simulink model "PowerSupplySimulation"  (R2015b)
settings: Solver=ode23t  StartTime=0.0  StopTime=5*T_mach  MaxStep=1e-7  MinStep=1e-9  RelTol=1e-3
undefined symbols (not defined in the file or in its folder): c2_val, Cs, delay_load, delayVC, den_c1, den_c2, duty_inv, duty_load, f_sw, I_ref, l1_val, l2_val, num_c1, num_c2, r_val, rc2_val, rl1_val, rl2_val, Rs, t2, T_mach, V_ref, Vd_val
libraries: powerlib x64, simulink x10, simulink_extras x6, powerlib_meascontrol x5
settings Model: Creator=Akshay  LastModifiedBy=Akshay
settings SolverCC: ZeroCrossAlgorithm=Adaptive
settings DataIOCC: SaveFormat=StructureWithTime
settings HardwareCC: ProdWordSize=32  ProdHWDeviceType=Specified

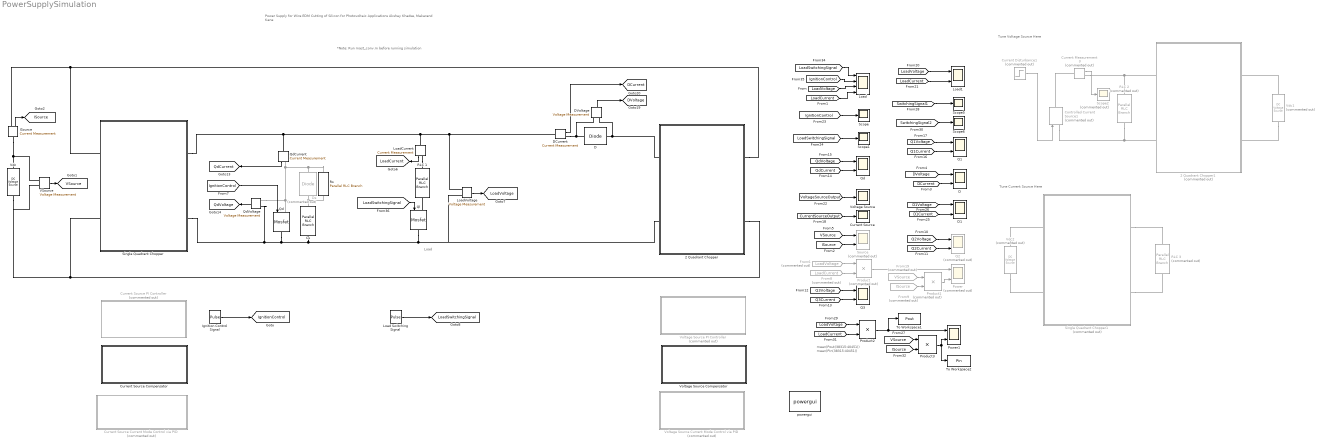
== system PowerSupplySimulation ==
  note: mean(Pout(38315:40451))
      | mean(Pin(38315:40451))
  note: Tune Current Source Here
  note: Tune Voltage Source Here
  note: Power Supply for Wire EDM Cutting of Silicon for Photovoltaic Applications
      |
      | Akshay Khadse, Makarand Kane
  note: Load
  note: *Note: Run mast_conv.m before running simulation
  " RLC 1" : powerlib/Elements/Parallel RLC Branch  LConnTagsString=a  RConnTagsString=__new0  BranchType=R  Resistance=r_val  Inductance=1e-3  SetiL0=off  InitialCurrent=0  Capacitance=0.1e-6  Setx0=off  InitialVoltage=0  Measurements=None
  " RLC 2" : powerlib/Elements/Parallel RLC Branch  Commented=on  LConnTagsString=a  RConnTagsString=__new0  BranchType=R  Resistance=r_val  Inductance=1e-3  SetiL0=off  InitialCurrent=0  Capacitance=0.1e-6  Setx0=off  InitialVoltage=0  Measurements=None
  " RLC 3" : powerlib/Elements/Parallel RLC Branch  Commented=on  LConnTagsString=a  RConnTagsString=__new0  BranchType=R  Resistance=r_val  Inductance=1e-3  SetiL0=off  InitialCurrent=0  Capacitance=0.1e-6  Setx0=off  InitialVoltage=0  Measurements=None
  " Rs" : powerlib/Elements/Parallel RLC Branch  LConnTagsString=a  RConnTagsString=__new0  BranchType=R  Resistance=Rs  Inductance=1e-3  SetiL0=off  InitialCurrent=0  Capacitance=0.1e-6  Setx0=off  InitialVoltage=0  Measurements=None
  2 Quadrant Chopper : Subsystem
  2 Quadrant Chopper1 : Subsystem  Commented=on
  Controlled Current Source1 : powerlib/Electrical Sources/Controlled Current Source  Commented=on  Initialize=on  Source_Type=AC  Amplitude=0  Phase=0  Frequency=0  Measurements=None
  Cs : powerlib/Elements/Parallel RLC Branch  LConnTagsString=a  RConnTagsString=__new0  BranchType=C  Resistance=r_val  Inductance=1e-3  SetiL0=off  InitialCurrent=0  Capacitance=Cs  Setx0=off  InitialVoltage=0  Measurements=None
  Current Disturbance1 : Step  Commented=on  Time=1e-3  After=10  SampleTime=0
  Current Measurement3 : powerlib/Measurements/Current Measurement  Commented=on  PhasorSimulation=off  OutputType=Complex  PSBequivalent=0
  Current Source : Scope
  Current Source Compensator : Subsystem
  Current Source Current Mode Control via PID : Subsystem  Commented=on
  Current Source PI Controller : Subsystem  Commented=on
  D : powerlib/Power Electronics/Diode  Ron=0.001  Lon=0  Vf=0.8  IC=0  UseSnubber=off  Rs=500  Cs=250e-9  Measurements=off
  "D " : Scope  NumInputPorts=2
  D1 : Scope  NumInputPorts=2
  DCurrent : powerlib/Measurements/Current Measurement  PhasorSimulation=off  OutputType=Complex  PSBequivalent=0
  DVoltage : powerlib/Measurements/Voltage Measurement  PhasorSimulation=off  OutputType=Complex  PSBequivalent=0
  Ds : powerlib/Power Electronics/Diode  Commented=on  Ron=0.001  Lon=0  Vf=0.8  IC=0  UseSnubber=off  Rs=500  Cs=250e-9  Measurements=off
  From19 : From  Commented=on  GotoTag=VSource  TagVisibility=global
  From6 : From  Commented=on  GotoTag=LoadVoltage  TagVisibility=global
  From8 : From  Commented=on  GotoTag=LoadCurrent  TagVisibility=global
  From9 : From  Commented=on  GotoTag=ISource  TagVisibility=global
  ISource : powerlib/Measurements/Current Measurement  PhasorSimulation=off  OutputType=Complex  PSBequivalent=0
  Ignition Control Signal : DiscretePulseGenerator  PulseType=Time based  Period=T_mach  PulseWidth=duty_inv  PhaseDelay=t2 + delayVC
  Load : Scope  NumInputPorts=4
  Load Switching Signal : DiscretePulseGenerator  PulseType=Time based  Period=T_mach  PulseWidth=duty_load  PhaseDelay=delay_load + delayVC
  Load1 : Scope  NumInputPorts=2
  LoadCurrent : powerlib/Measurements/Current Measurement  PhasorSimulation=off  OutputType=Complex  PSBequivalent=0
  LoadVoltage : powerlib/Measurements/Voltage Measurement  PhasorSimulation=off  OutputType=Complex  PSBequivalent=0
  Power : Scope  Commented=on  NumInputPorts=2
  Power1 : Scope  NumInputPorts=2
  Product : Product  Commented=on
  Product1 : Product  Commented=on
  Product2 : Product
  Product3 : Product
  "Q1 " : Scope  NumInputPorts=2
  "Q2 " : Scope  Commented=on  NumInputPorts=2
  "Q3 " : Scope  NumInputPorts=2
  Qd : powerlib/Power Electronics/Mosfet  Ron=0.1  Lon=0  Rd=0.01  Vfd=0  IC=0  Rs=1e5  Cs=inf  Measurements=off
  "Qd " : Scope  NumInputPorts=2
  QdCurrent : powerlib/Measurements/Current Measurement  PhasorSimulation=off  OutputType=Complex  PSBequivalent=0
  QdVoltage : powerlib/Measurements/Voltage Measurement  PhasorSimulation=off  OutputType=Complex  PSBequivalent=0
  Ql : powerlib/Power Electronics/Mosfet  Ron=0.1  Lon=0  Rd=0.01  Vfd=0  IC=0  Rs=1e5  Cs=inf  Measurements=off
  Scope{,1,5..6} (4 alike) : Scope
  Scope2 : Scope  Commented=on
  Single Quadrant Chopper : Subsystem
  Single Quadrant Chopper1 : Subsystem  Commented=on
  Source : Scope  Commented=on  NumInputPorts=2
  To Workspace1 : ToWorkspace  VariableName=Pout  SampleTime=-1
  To Workspace2 : ToWorkspace  VariableName=Pin  SampleTime=-1
  VSource : powerlib/Measurements/Voltage Measurement  PhasorSimulation=off  OutputType=Complex  PSBequivalent=0
  Vdc : powerlib/Electrical Sources/DC Voltage Source  Amplitude=Vd_val  Measurements=Voltage
  Vdc1 : powerlib/Electrical Sources/DC Voltage Source  Commented=on  Amplitude=Vd_val  Measurements=Voltage
  Vdc2 : powerlib/Electrical Sources/DC Voltage Source  Commented=on  Amplitude=Vd_val  Measurements=Voltage
  Voltage Source : Scope
  Voltage Source Compensator : Subsystem
  Voltage Source Current Mode Control via PID : Subsystem  Commented=on
  Voltage Source PI Controller : Subsystem  Commented=on
  powergui : powerlib/powergui  Priority=1  SimulationMode=Continuous  SolverType=Backward Euler  SampleTime=5e-07  frequency=60  SPID=on  DisableSnubberDevices=off  DisableRonSwitches=off  DisableVfSwitches=off  SwTol=0  DisplayEquations=off  Interpol=off  ExternalGateDelay=off  methode=off  Ts=0  FunctionMessages=off  echomessages=off  HookPort=off  EnableUseOfTLC=off  x0status=zero  frequencyindice=0  Pbase=100e6  ErrMax=1e-4  Iterations=50  UnitsV=kV  UnitsW=MW  buscounter=0  RestoreLinks=warning  ResistiveCurrentMeasurement=off  Frange=[0:2:500]  Ylog=off  Xlog=on  ShowGrid=off  save=off  variable=ZData  structure=ScopeData  ZoomFFT=off  StartTime=0.0  cycles=5  DisplayStyle=2  fundamental=50  FreqAxis=off  MaxFrequency=50000  frequencyindicesteady=1  RmsSteady=1  display=off
  tag scope: DCurrent=global, DVoltage=global, ISource=global, IgnitionControl=global, LoadCurrent=global, LoadSwitchingSignal=global, LoadVoltage=global, QdCurrent=global, QdVoltage=global, VSource=global
  wires:
  Ignition Control Signal/1 -> [IgnitionControl]
  Load Switching Signal/1 -> [LoadSwitchingSignal]
  [Q2Voltage] -> "Q2 "/1
  [Q2Current] -> "Q2 "/2
  [Q1Voltage] -> "Q1 "/1
  [Q1Current] -> "Q1 "/2
  [QdVoltage] -> "Qd "/1
  [QdCurrent] -> "Qd "/2
  [VoltageSourceOutput] -> Voltage Source/1
  [IgnitionControl] -> Scope/1
  [LoadSwitchingSignal] -> Scope1/1
  [CurrentSourceOutput] -> Current Source/1
  LoadCurrent/1 -> [LoadCurrent]
  LoadVoltage/1 -> [LoadVoltage]
  [IgnitionControl] -> Qd/1
  QdCurrent/1 -> [QdCurrent]
  QdVoltage/1 -> [QdVoltage]
  DVoltage/1 -> [DVoltage]
  DCurrent/1 -> [DCurrent]
  [LoadSwitchingSignal] -> Load/1
  [IgnitionControl] -> Load/2
  [LoadVoltage] -> Load/3
  [LoadCurrent] -> Load/4
  [LoadSwitchingSignal] -> Ql/1
  [SwitchingSignal2] -> Scope6/1
  [SwitchingSignal1] -> Scope5/1
  [DVoltage] -> "D "/1
  [DCurrent] -> "D "/2
  VSource/1 -> [VSource]
  ISource/1 -> [ISource]
  [VSource] -> Source/1
  [ISource] -> Source/2
  From6/1 -> Product/1
  From8/1 -> Product/2
  From19/1 -> Product1/1
  From9/1 -> Product1/2
  Product/1 -> Power/1
  Product1/1 -> Power/2
  [D1Voltage] -> D1/1
  [D1Current] -> D1/2
  Current Disturbance1/1 -> Controlled Current Source1/1
  Current Measurement3/1 -> Scope2/1
  [LoadVoltage] -> Load1/1
  [LoadCurrent] -> Load1/2
  [Q3Voltage] -> "Q3 "/1
  [Q3Current] -> "Q3 "/2
  [LoadVoltage] -> Product2/1
  [LoadCurrent] -> Product2/2
  [VSource] -> Product3/1
  [ISource] -> Product3/2
  Product2/1 -> To Workspace1/1, Power1/1
  Product3/1 -> Power1/2, To Workspace2/1
  connections:
  LoadCurrent/RConn1 -- " RLC 1"/LConn1
  Ds/LConn1 -- QdVoltage/LConn1 -- Qd/LConn1 -- QdCurrent/RConn1 -- " Rs"/LConn1
  DVoltage/LConn1 -- DCurrent/RConn1 -- D/LConn1
  DCurrent/LConn1 -- LoadVoltage/LConn1 -- LoadCurrent/LConn1 -- QdCurrent/LConn1 -- Single Quadrant Chopper/RConn1
  2 Quadrant Chopper/RConn1 -- ISource/RConn1 -- Single Quadrant Chopper/LConn1
  2 Quadrant Chopper/RConn2 -- VSource/LConn2 -- Vdc/LConn1 -- Single Quadrant Chopper/LConn2
  Ql/LConn1 -- " RLC 1"/RConn1
  D/RConn1 -- 2 Quadrant Chopper/LConn1 -- DVoltage/LConn2
  Qd/RConn1 -- 2 Quadrant Chopper/LConn2 -- LoadVoltage/LConn2 -- Ql/RConn1 -- Cs/RConn1 -- QdVoltage/LConn2 -- Single Quadrant Chopper/RConn2
  ISource/LConn1 -- Vdc/RConn1 -- VSource/LConn1
  " RLC 2"/LConn1 -- Current Measurement3/RConn1 -- 2 Quadrant Chopper1/LConn1
  " RLC 2"/RConn1 -- Controlled Current Source1/LConn1 -- 2 Quadrant Chopper1/LConn2
  Vdc1/RConn1 -- 2 Quadrant Chopper1/RConn1
  Vdc1/LConn1 -- 2 Quadrant Chopper1/RConn2
  Vdc2/RConn1 -- Single Quadrant Chopper1/LConn1
  Vdc2/LConn1 -- Single Quadrant Chopper1/LConn2
  Single Quadrant Chopper1/RConn1 -- " RLC 3"/LConn1
  Single Quadrant Chopper1/RConn2 -- " RLC 3"/RConn1
  Ds/RConn1 -- " Rs"/RConn1 -- Cs/LConn1
  Controlled Current Source1/RConn1 -- Current Measurement3/LConn1

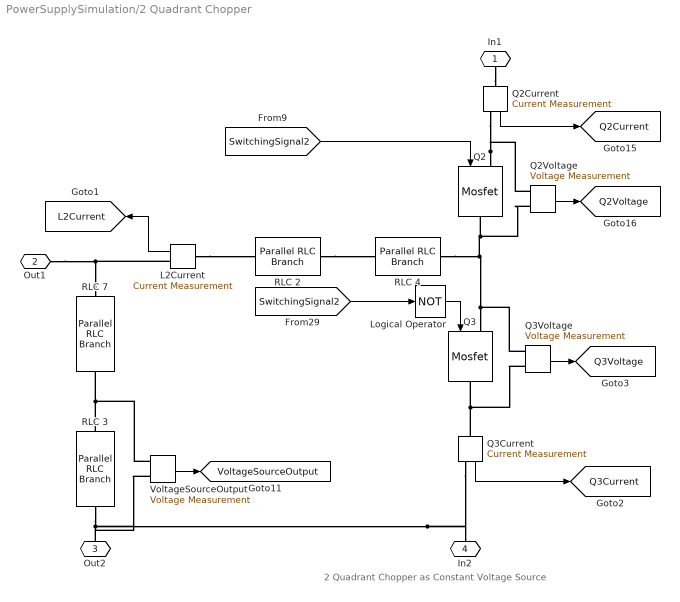
== system PowerSupplySimulation/2 Quadrant Chopper ==
  note: 2 Quadrant Chopper as Constant Voltage Source
  " RLC 2" : powerlib/Elements/Parallel RLC Branch  LConnTagsString=a  RConnTagsString=__new0  BranchType=R  Resistance=rl2_val  Inductance=5e-6  SetiL0=off  InitialCurrent=0  Capacitance=0.3e-6  Setx0=off  InitialVoltage=0  Measurements=None
  " RLC 3" : powerlib/Elements/Parallel RLC Branch  LConnTagsString=a  RConnTagsString=__new0  BranchType=C  Resistance=1  Inductance=1e-3  SetiL0=off  InitialCurrent=0  Capacitance=c2_val  Setx0=off  InitialVoltage=50  Measurements=None
  " RLC 4" : powerlib/Elements/Parallel RLC Branch  LConnTagsString=a  RConnTagsString=__new0  BranchType=L  Resistance=50  Inductance=l2_val  SetiL0=off  InitialCurrent=0  Capacitance=0.3e-6  Setx0=off  InitialVoltage=0  Measurements=None
  " RLC 7" : powerlib/Elements/Parallel RLC Branch  LConnTagsString=a  RConnTagsString=__new0  BranchType=R  Resistance=rc2_val  Inductance=1e-3  SetiL0=off  InitialCurrent=0  Capacitance=0.1e-6  Setx0=off  InitialVoltage=0  Measurements=None
  L2Current : powerlib/Measurements/Current Measurement  PhasorSimulation=off  OutputType=Complex  PSBequivalent=0
  Logical Operator : Logic  Operator=NOT  AllPortsSameDT=off  OutDataTypeStr=boolean
  Q2 : powerlib/Power Electronics/Mosfet  Ron=0.1  Lon=0  Rd=0.01  Vfd=0  IC=0  Rs=1e5  Cs=inf  Measurements=off
  Q2Current : powerlib/Measurements/Current Measurement  PhasorSimulation=off  OutputType=Complex  PSBequivalent=0
  Q2Voltage : powerlib/Measurements/Voltage Measurement  PhasorSimulation=off  OutputType=Complex  PSBequivalent=0
  Q3 : powerlib/Power Electronics/Mosfet  Ron=0.1  Lon=0  Rd=0.01  Vfd=0  IC=0  Rs=1e5  Cs=inf  Measurements=off
  Q3Current : powerlib/Measurements/Current Measurement  PhasorSimulation=off  OutputType=Complex  PSBequivalent=0
  Q3Voltage : powerlib/Measurements/Voltage Measurement  PhasorSimulation=off  OutputType=Complex  PSBequivalent=0
  VoltageSourceOutput : powerlib/Measurements/Voltage Measurement  PhasorSimulation=off  OutputType=Complex  PSBequivalent=0
  In1 : PMIOPort  Port=1  Side=Right
  Out1 : PMIOPort  Port=2  Side=Left
  Out2 : PMIOPort  Port=3  Side=Left
  In2 : PMIOPort  Port=4  Side=Right
  tag scope: L2Current=global, Q2Current=global, Q2Voltage=global, Q3Current=global, Q3Voltage=global, VoltageSourceOutput=global
  wires:
  Logical Operator/1 -> Q3/1
  VoltageSourceOutput/1 -> [VoltageSourceOutput]
  Q3Current/1 -> [Q3Current]
  Q3Voltage/1 -> [Q3Voltage]
  Q2Voltage/1 -> [Q2Voltage]
  Q2Current/1 -> [Q2Current]
  [SwitchingSignal2] -> Q2/1
  [SwitchingSignal2] -> Logical Operator/1
  L2Current/1 -> [L2Current]
  connections:
  " RLC 3"/RConn1 -- VoltageSourceOutput/LConn2 -- Q3Current/RConn1 -- In2/RConn1 -- Out2/RConn1
  VoltageSourceOutput/LConn1 -- " RLC 3"/LConn1 -- " RLC 7"/RConn1
  Q3Voltage/LConn2 -- Q3Current/LConn1 -- Q3/RConn1
  Q2/LConn1 -- Q2Voltage/LConn1 -- Q2Current/RConn1
  " RLC 2"/RConn1 -- " RLC 4"/LConn1
  In1/RConn1 -- Q2Current/LConn1
  Out1/RConn1 -- L2Current/RConn1 -- " RLC 7"/LConn1
  " RLC 4"/RConn1 -- Q3Voltage/LConn1 -- Q3/LConn1 -- Q2Voltage/LConn2 -- Q2/RConn1
  L2Current/LConn1 -- " RLC 2"/LConn1

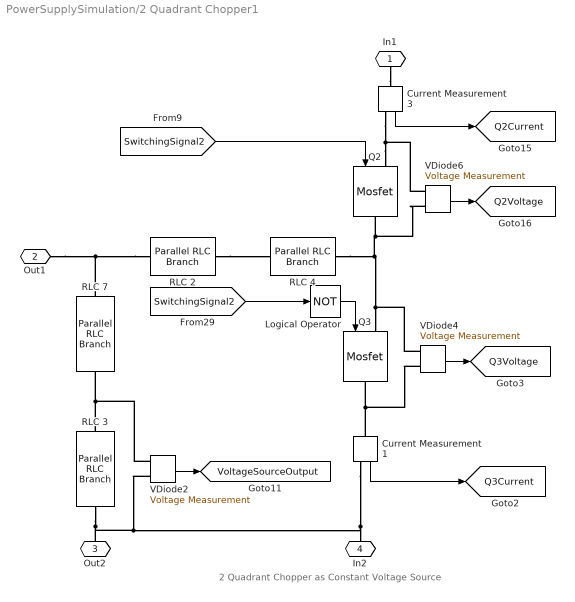
== system PowerSupplySimulation/2 Quadrant Chopper1 ==
  note: 2 Quadrant Chopper as Constant Voltage Source
  " RLC 2" : powerlib/Elements/Parallel RLC Branch  LConnTagsString=a  RConnTagsString=__new0  BranchType=R  Resistance=rl2_val  Inductance=5e-6  SetiL0=off  InitialCurrent=0  Capacitance=0.3e-6  Setx0=off  InitialVoltage=0  Measurements=None
  " RLC 3" : powerlib/Elements/Parallel RLC Branch  LConnTagsString=a  RConnTagsString=__new0  BranchType=C  Resistance=1  Inductance=1e-3  SetiL0=off  InitialCurrent=0  Capacitance=c2_val  Setx0=off  InitialVoltage=50  Measurements=None
  " RLC 4" : powerlib/Elements/Parallel RLC Branch  LConnTagsString=a  RConnTagsString=__new0  BranchType=L  Resistance=50  Inductance=l2_val  SetiL0=off  InitialCurrent=0  Capacitance=0.3e-6  Setx0=off  InitialVoltage=0  Measurements=None
  " RLC 7" : powerlib/Elements/Parallel RLC Branch  LConnTagsString=a  RConnTagsString=__new0  BranchType=R  Resistance=rc2_val  Inductance=1e-3  SetiL0=off  InitialCurrent=0  Capacitance=0.1e-6  Setx0=off  InitialVoltage=0  Measurements=None
  Current Measurement1 : powerlib/Measurements/Current Measurement  PhasorSimulation=off  OutputType=Complex  PSBequivalent=0
  Current Measurement3 : powerlib/Measurements/Current Measurement  PhasorSimulation=off  OutputType=Complex  PSBequivalent=0
  Logical Operator : Logic  Operator=NOT  AllPortsSameDT=off  OutDataTypeStr=boolean
  Q2 : powerlib/Power Electronics/Mosfet  Ron=0.1  Lon=0  Rd=0.01  Vfd=0  IC=0  Rs=1e5  Cs=inf  Measurements=off
  Q3 : powerlib/Power Electronics/Mosfet  Ron=0.1  Lon=0  Rd=0.01  Vfd=0  IC=0  Rs=1e5  Cs=inf  Measurements=off
  VDiode2 : powerlib/Measurements/Voltage Measurement  PhasorSimulation=off  OutputType=Complex  PSBequivalent=0
  VDiode4 : powerlib/Measurements/Voltage Measurement  PhasorSimulation=off  OutputType=Complex  PSBequivalent=0
  VDiode6 : powerlib/Measurements/Voltage Measurement  PhasorSimulation=off  OutputType=Complex  PSBequivalent=0
  In1 : PMIOPort  Port=1  Side=Right
  Out1 : PMIOPort  Port=2  Side=Left
  Out2 : PMIOPort  Port=3  Side=Left
  In2 : PMIOPort  Port=4  Side=Right
  tag scope: Q2Current=global, Q2Voltage=global, Q3Current=global, Q3Voltage=global, VoltageSourceOutput=global
  wires:
  Logical Operator/1 -> Q3/1
  VDiode2/1 -> [VoltageSourceOutput]
  Current Measurement1/1 -> [Q3Current]
  VDiode4/1 -> [Q3Voltage]
  VDiode6/1 -> [Q2Voltage]
  Current Measurement3/1 -> [Q2Current]
  [SwitchingSignal2] -> Q2/1
  [SwitchingSignal2] -> Logical Operator/1
  connections:
  " RLC 3"/RConn1 -- Current Measurement1/RConn1 -- In2/RConn1 -- VDiode2/LConn2 -- Out2/RConn1
  VDiode2/LConn1 -- " RLC 3"/LConn1 -- " RLC 7"/RConn1
  VDiode4/LConn2 -- Current Measurement1/LConn1 -- Q3/RConn1
  Q2/LConn1 -- VDiode6/LConn1 -- Current Measurement3/RConn1
  " RLC 2"/RConn1 -- " RLC 4"/LConn1
  In1/RConn1 -- Current Measurement3/LConn1
  " RLC 2"/LConn1 -- " RLC 7"/LConn1 -- Out1/RConn1
  " RLC 4"/RConn1 -- VDiode4/LConn1 -- Q3/LConn1 -- VDiode6/LConn2 -- Q2/RConn1

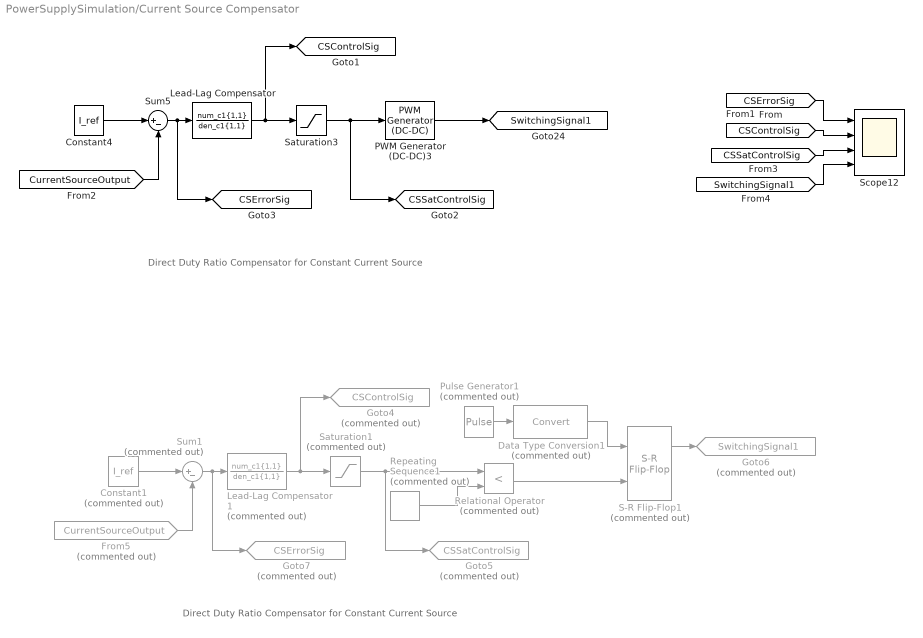
== system PowerSupplySimulation/Current Source Compensator ==
  note: Direct Duty Ratio Compensator for Constant Current Source
  note: Direct Duty Ratio Compensator for Constant Current Source
  Constant1 : Constant  Commented=on  Value=I_ref
  Constant4 : Constant  Value=I_ref
  Data Type Conversion1 : DataTypeConversion  Commented=on
  From5 : From  Commented=on  GotoTag=CurrentSourceOutput  TagVisibility=global
  Goto4 : Goto  Commented=on  GotoTag=CSControlSig  TagVisibility=global
  Goto5 : Goto  Commented=on  GotoTag=CSSatControlSig  TagVisibility=global
  Goto6 : Goto  Commented=on  GotoTag=SwitchingSignal1  TagVisibility=global
  Goto7 : Goto  Commented=on  GotoTag=CSErrorSig  TagVisibility=global
  Lead-Lag Compensator : TransferFcn  Numerator=num_c1{1,1}  Denominator=den_c1{1,1}
  Lead-Lag Compensator1 : TransferFcn  Commented=on  Numerator=num_c1{1,1}  Denominator=den_c1{1,1}
  PWM Generator (DC-DC)3 : powerlib_meascontrol/Pulse & Signal Generators/PWM Generator (DC-DC)  Fsw=f_sw  Ts=0
  Pulse Generator1 : DiscretePulseGenerator  Commented=on  PulseType=Time based  Period=1/f_sw  PulseWidth=5
  Relational Operator : RelationalOperator  Commented=on  Operator=<  OutDataTypeStr=boolean
  Repeating Sequence1 : simulink/Sources/Repeating Sequence  Commented=on  rep_seq_t=[0 1/f_sw]  rep_seq_y=[0 1]
  S-R Flip-Flop1 : simulink_extras/Flip Flops/S-R Flip-Flop  Commented=on  initial_condition=0
  Saturation1 : Saturate  Commented=on  UpperLimit=0.99  LowerLimit=0
  Saturation3 : Saturate  UpperLimit=0.99  LowerLimit=0
  Scope12 : Scope  NumInputPorts=4
  Sum1 : Sum  Commented=on  Inputs=|+-
  Sum5 : Sum  Inputs=|+-
  tag scope: CSControlSig=global, CSErrorSig=global, CSSatControlSig=global, SwitchingSignal1=global
  wires:
  Sum5/1 -> [CSErrorSig], Lead-Lag Compensator/1
  Constant4/1 -> Sum5/1
  [CurrentSourceOutput] -> Sum5/2
  Lead-Lag Compensator/1 -> Saturation3/1, [CSControlSig]
  Saturation3/1 -> [CSSatControlSig], PWM Generator (DC-DC)3/1
  PWM Generator (DC-DC)3/1 -> [SwitchingSignal1]
  [CSErrorSig] -> Scope12/1
  [CSControlSig] -> Scope12/2
  [CSSatControlSig] -> Scope12/3
  [SwitchingSignal1] -> Scope12/4
  Sum1/1 -> Goto7/1, Lead-Lag Compensator1/1
  Constant1/1 -> Sum1/1
  From5/1 -> Sum1/2
  Lead-Lag Compensator1/1 -> Saturation1/1, Goto4/1
  Saturation1/1 -> Relational Operator/1, Goto5/1
  Repeating Sequence1/1 -> Relational Operator/2
  S-R Flip-Flop1/1 -> Goto6/1
  Pulse Generator1/1 -> Data Type Conversion1/1
  Data Type Conversion1/1 -> S-R Flip-Flop1/1
  Relational Operator/1 -> S-R Flip-Flop1/2

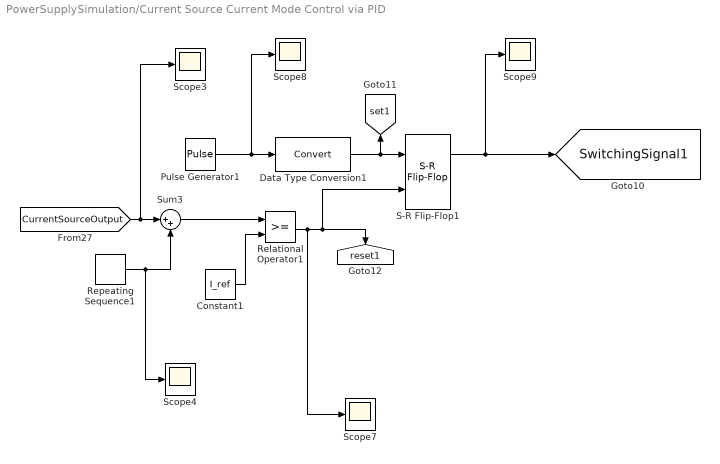
== system PowerSupplySimulation/Current Source Current Mode Control via PID ==
  Constant1 : Constant  Value=I_ref
  Data Type Conversion1 : DataTypeConversion
  Pulse Generator1 : DiscretePulseGenerator  PulseType=Time based  Period=1/f_sw  PulseWidth=5
  Relational Operator1 : RelationalOperator  OutDataTypeStr=boolean
  Repeating Sequence1 : simulink/Sources/Repeating Sequence  rep_seq_t=[0 1/f_sw]  rep_seq_y=[0 0]
  S-R Flip-Flop1 : simulink_extras/Flip Flops/S-R Flip-Flop  initial_condition=0
  Scope{3..4,7..9} (5 alike) : Scope
  Sum3 : Sum  Inputs=|++
  tag scope: SwitchingSignal1=global, reset1=global, set1=global
  wires:
  Pulse Generator1/1 -> Scope8/1, Data Type Conversion1/1
  Data Type Conversion1/1 -> S-R Flip-Flop1/1, [set1]
  Relational Operator1/1 -> Scope7/1, S-R Flip-Flop1/2, [reset1]
  S-R Flip-Flop1/1 -> Scope9/1, [SwitchingSignal1]
  [CurrentSourceOutput] -> Scope3/1, Sum3/1
  Repeating Sequence1/1 -> Scope4/1, Sum3/2
  Sum3/1 -> Relational Operator1/1
  Constant1/1 -> Relational Operator1/2

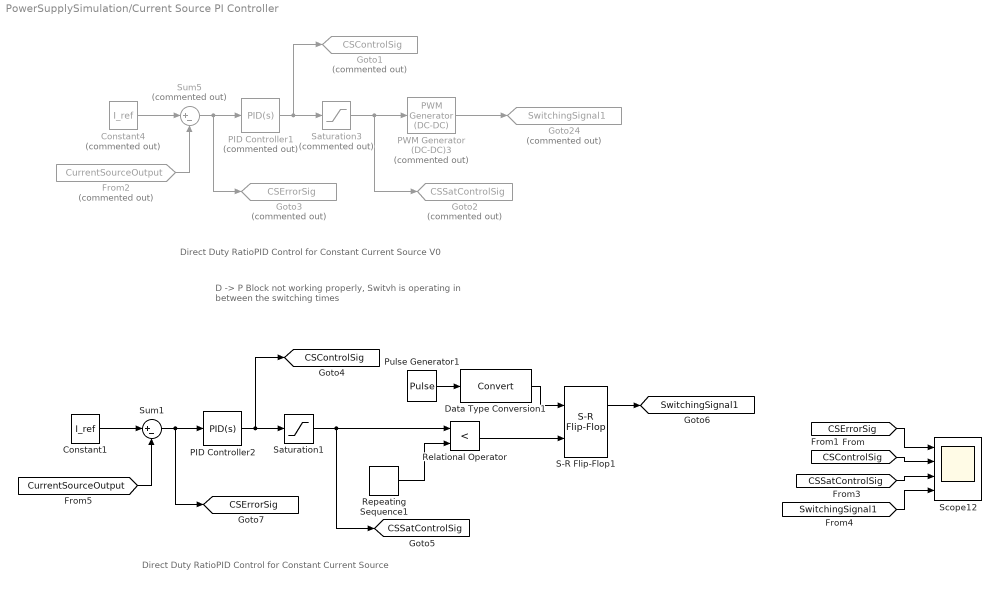
== system PowerSupplySimulation/Current Source PI Controller ==
  note: D -> P Block not working properly,
      | Switvh is operating in between the switching times
  note: Direct Duty RatioPID Control for Constant Current Source V0
  note: Direct Duty RatioPID Control for Constant Current Source
  Constant1 : Constant  Value=I_ref
  Constant4 : Constant  Commented=on  Value=I_ref
  Data Type Conversion1 : DataTypeConversion
  From2 : From  Commented=on  GotoTag=CurrentSourceOutput  TagVisibility=global
  Goto1 : Goto  Commented=on  GotoTag=CSControlSig  TagVisibility=global
  Goto2 : Goto  Commented=on  GotoTag=CSSatControlSig  TagVisibility=global
  Goto24 : Goto  Commented=on  GotoTag=SwitchingSignal1  TagVisibility=global
  Goto3 : Goto  Commented=on  GotoTag=CSErrorSig  TagVisibility=global
  PID Controller1 : simulink/Continuous/PID Controller  Commented=on  Controller=PID  TimeDomain=Continuous-time  SampleTime=-1  IntegratorMethod=Forward Euler  FilterMethod=Forward Euler  Form=Parallel  UseFilter=on  ControllerParametersSource=internal  P=3  I=0  D=0  N=5  InitialConditionSource=internal  InitialConditionForIntegrator=0  InitialConditionForFilter=0  ExternalReset=none  LimitOutput=off  UpperSaturationLimit=inf  LowerSaturationLimit=-inf  LinearizeAsGain=on  AntiWindupMode=none  Kb=1  TrackingMode=off  Kt=1  PParamMin=[]  PParamMax=[]  IParamMin=[]  IParamMax=[]  DParamMin=[]  DParamMax=[]  NParamMin=[]  NParamMax=[]  KbParamMin=[]  KbParamMax=[]  KtParamMin=[]  KtParamMax=[]  POutMin=[]  POutMax=[]  IOutMin=[]  IOutMax=[]  DOutMin=[]  DOutMax=[]  NOutMin=[]  NOutMax=[]  KbOutMin=[]  KbOutMax=[]  KtOutMin=[]  KtOutMax=[]  IntegratorOutMin=[]  IntegratorOutMax=[]  FilterOutMin=[]  FilterOutMax=[]  SumOutMin=[]  SumOutMax=[]  SumI1OutMin=[]  SumI1OutMax=[]  SumI2OutMin=[]  SumI2OutMax=[]  SumI3OutMin=[]  SumI3OutMax=[]  SumDOutMin=[]  SumDOutMax=[]  SaturationOutMin=[]  SaturationOutMax=[]  IntegratorContinuousStateAttributes=''  IntegratorStateMustResolveToSignalObject=off  IntegratorRTWStateStorageClass=Auto  FilterContinuousStateAttributes=''  FilterStateMustResolveToSignalObject=off  FilterRTWStateStorageClass=Auto  DifferentiatorICPrevScaledInput=0  DifferentiatorOutMin=[]  DifferentiatorOutMax=[]
  PID Controller2 : simulink/Continuous/PID Controller  Controller=PID  TimeDomain=Continuous-time  SampleTime=-1  IntegratorMethod=Forward Euler  FilterMethod=Forward Euler  Form=Parallel  UseFilter=on  ControllerParametersSource=internal  P=1  I=0  D=0  N=5  InitialConditionSource=internal  InitialConditionForIntegrator=0  InitialConditionForFilter=0  ExternalReset=none  LimitOutput=off  UpperSaturationLimit=inf  LowerSaturationLimit=-inf  LinearizeAsGain=on  AntiWindupMode=none  Kb=1  TrackingMode=off  Kt=1  PParamMin=[]  PParamMax=[]  IParamMin=[]  IParamMax=[]  DParamMin=[]  DParamMax=[]  NParamMin=[]  NParamMax=[]  KbParamMin=[]  KbParamMax=[]  KtParamMin=[]  KtParamMax=[]  POutMin=[]  POutMax=[]  IOutMin=[]  IOutMax=[]  DOutMin=[]  DOutMax=[]  NOutMin=[]  NOutMax=[]  KbOutMin=[]  KbOutMax=[]  KtOutMin=[]  KtOutMax=[]  IntegratorOutMin=[]  IntegratorOutMax=[]  FilterOutMin=[]  FilterOutMax=[]  SumOutMin=[]  SumOutMax=[]  SumI1OutMin=[]  SumI1OutMax=[]  SumI2OutMin=[]  SumI2OutMax=[]  SumI3OutMin=[]  SumI3OutMax=[]  SumDOutMin=[]  SumDOutMax=[]  SaturationOutMin=[]  SaturationOutMax=[]  IntegratorContinuousStateAttributes=''  IntegratorStateMustResolveToSignalObject=off  IntegratorRTWStateStorageClass=Auto  FilterContinuousStateAttributes=''  FilterStateMustResolveToSignalObject=off  FilterRTWStateStorageClass=Auto  DifferentiatorICPrevScaledInput=0  DifferentiatorOutMin=[]  DifferentiatorOutMax=[]
  PWM Generator (DC-DC)3 : powerlib_meascontrol/Pulse & Signal Generators/PWM Generator (DC-DC)  Commented=on  Fsw=f_sw  Ts=0
  Pulse Generator1 : DiscretePulseGenerator  PulseType=Time based  Period=1/f_sw  PulseWidth=5
  Relational Operator : RelationalOperator  Operator=<  OutDataTypeStr=boolean
  Repeating Sequence1 : simulink/Sources/Repeating Sequence  rep_seq_t=[0 1/f_sw]  rep_seq_y=[0 1]
  S-R Flip-Flop1 : simulink_extras/Flip Flops/S-R Flip-Flop  initial_condition=0
  Saturation1 : Saturate  UpperLimit=0.99  LowerLimit=0
  Saturation3 : Saturate  Commented=on  UpperLimit=0.99  LowerLimit=0
  Scope12 : Scope  NumInputPorts=4
  Sum1 : Sum  Inputs=|+-
  Sum5 : Sum  Commented=on  Inputs=|+-
  tag scope: CSControlSig=global, CSErrorSig=global, CSSatControlSig=global, SwitchingSignal1=global
  wires:
  Sum5/1 -> Goto3/1, PID Controller1/1
  Constant4/1 -> Sum5/1
  From2/1 -> Sum5/2
  PID Controller1/1 -> Saturation3/1, Goto1/1
  Saturation3/1 -> Goto2/1, PWM Generator (DC-DC)3/1
  PWM Generator (DC-DC)3/1 -> Goto24/1
  [CSErrorSig] -> Scope12/1
  [CSControlSig] -> Scope12/2
  [CSSatControlSig] -> Scope12/3
  [SwitchingSignal1] -> Scope12/4
  Sum1/1 -> [CSErrorSig], PID Controller2/1
  Constant1/1 -> Sum1/1
  [CurrentSourceOutput] -> Sum1/2
  PID Controller2/1 -> Saturation1/1, [CSControlSig]
  Repeating Sequence1/1 -> Relational Operator/2
  Relational Operator/1 -> S-R Flip-Flop1/2
  Saturation1/1 -> Relational Operator/1, [CSSatControlSig]
  S-R Flip-Flop1/1 -> [SwitchingSignal1]
  Data Type Conversion1/1 -> S-R Flip-Flop1/1
  Pulse Generator1/1 -> Data Type Conversion1/1

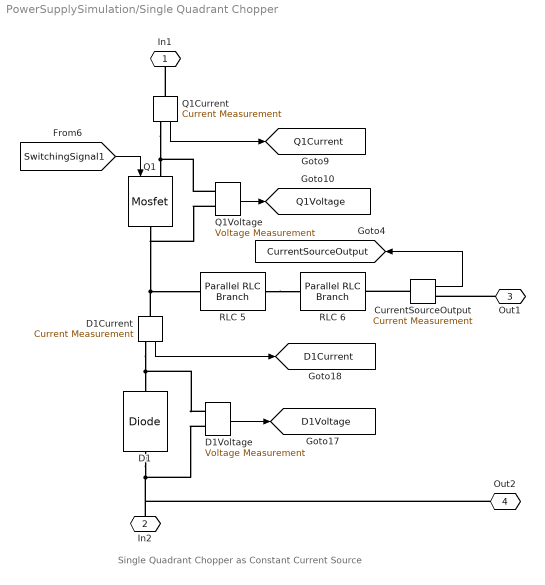
== system PowerSupplySimulation/Single Quadrant Chopper ==
  note: Single Quadrant Chopper as Constant Current Source
  " RLC 5" : powerlib/Elements/Parallel RLC Branch  LConnTagsString=a  RConnTagsString=__new0  BranchType=R  Resistance=rl1_val  Inductance=5e-6  SetiL0=off  InitialCurrent=0  Capacitance=0.3e-6  Setx0=off  InitialVoltage=0  Measurements=None
  " RLC 6" : powerlib/Elements/Parallel RLC Branch  LConnTagsString=a  RConnTagsString=__new0  BranchType=L  Resistance=50  Inductance=l1_val  SetiL0=off  InitialCurrent=100  Capacitance=0.3e-6  Setx0=off  InitialVoltage=0  Measurements=None
  CurrentSourceOutput : powerlib/Measurements/Current Measurement  PhasorSimulation=off  OutputType=Complex  PSBequivalent=0
  D1 : powerlib/Power Electronics/Diode  Ron=0.001  Lon=0  Vf=0.8  IC=0  UseSnubber=off  Rs=500  Cs=250e-9  Measurements=off
  D1Current : powerlib/Measurements/Current Measurement  PhasorSimulation=off  OutputType=Complex  PSBequivalent=0
  D1Voltage : powerlib/Measurements/Voltage Measurement  PhasorSimulation=off  OutputType=Complex  PSBequivalent=0
  Q1 : powerlib/Power Electronics/Mosfet  Ron=0.1  Lon=0  Rd=0.01  Vfd=0  IC=0  Rs=1e5  Cs=inf  Measurements=off
  Q1Current : powerlib/Measurements/Current Measurement  PhasorSimulation=off  OutputType=Complex  PSBequivalent=0
  Q1Voltage : powerlib/Measurements/Voltage Measurement  PhasorSimulation=off  OutputType=Complex  PSBequivalent=0
  In1 : PMIOPort  Port=1  Side=Left
  In2 : PMIOPort  Port=2  Side=Left
  Out1 : PMIOPort  Port=3  Side=Right
  Out2 : PMIOPort  Port=4  Side=Right
  tag scope: CurrentSourceOutput=global, D1Current=global, D1Voltage=global, Q1Current=global, Q1Voltage=global
  wires:
  CurrentSourceOutput/1 -> [CurrentSourceOutput]
  [SwitchingSignal1] -> Q1/1
  Q1Current/1 -> [Q1Current]
  Q1Voltage/1 -> [Q1Voltage]
  D1Current/1 -> [D1Current]
  D1Voltage/1 -> [D1Voltage]
  connections:
  Q1Voltage/LConn2 -- Q1/RConn1 -- D1Current/LConn1 -- " RLC 5"/LConn1
  Q1Current/LConn1 -- In1/RConn1
  " RLC 5"/RConn1 -- " RLC 6"/LConn1
  CurrentSourceOutput/LConn1 -- " RLC 6"/RConn1
  Q1Current/RConn1 -- Q1Voltage/LConn1 -- Q1/LConn1
  D1Current/RConn1 -- D1/RConn1 -- D1Voltage/LConn1
  D1Voltage/LConn2 -- In2/RConn1 -- Out2/RConn1 -- D1/LConn1
  Out1/RConn1 -- CurrentSourceOutput/RConn1

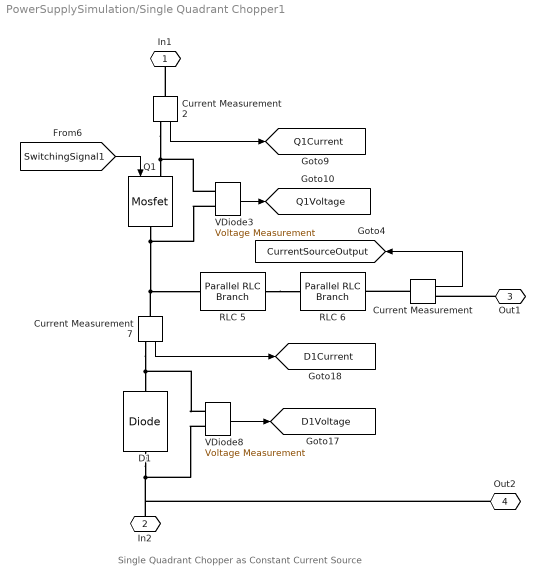
== system PowerSupplySimulation/Single Quadrant Chopper1 ==
  note: Single Quadrant Chopper as Constant Current Source
  " RLC 5" : powerlib/Elements/Parallel RLC Branch  LConnTagsString=a  RConnTagsString=__new0  BranchType=R  Resistance=rl1_val  Inductance=5e-6  SetiL0=off  InitialCurrent=0  Capacitance=0.3e-6  Setx0=off  InitialVoltage=0  Measurements=None
  " RLC 6" : powerlib/Elements/Parallel RLC Branch  LConnTagsString=a  RConnTagsString=__new0  BranchType=L  Resistance=50  Inductance=l1_val  SetiL0=off  InitialCurrent=100  Capacitance=0.3e-6  Setx0=off  InitialVoltage=0  Measurements=None
  Current Measurement2 : powerlib/Measurements/Current Measurement  PhasorSimulation=off  OutputType=Complex  PSBequivalent=0
  Current Measurement7 : powerlib/Measurements/Current Measurement  PhasorSimulation=off  OutputType=Complex  PSBequivalent=0
  Current Measurement : powerlib/Measurements/Current Measurement  PhasorSimulation=off  OutputType=Complex  PSBequivalent=0
  D1 : powerlib/Power Electronics/Diode  Ron=0.001  Lon=0  Vf=0.8  IC=0  UseSnubber=off  Rs=500  Cs=250e-9  Measurements=off
  Q1 : powerlib/Power Electronics/Mosfet  Ron=0.1  Lon=0  Rd=0.01  Vfd=0  IC=0  Rs=1e5  Cs=inf  Measurements=off
  VDiode3 : powerlib/Measurements/Voltage Measurement  PhasorSimulation=off  OutputType=Complex  PSBequivalent=0
  VDiode8 : powerlib/Measurements/Voltage Measurement  PhasorSimulation=off  OutputType=Complex  PSBequivalent=0
  In1 : PMIOPort  Port=1  Side=Left
  In2 : PMIOPort  Port=2  Side=Left
  Out1 : PMIOPort  Port=3  Side=Right
  Out2 : PMIOPort  Port=4  Side=Right
  tag scope: CurrentSourceOutput=global, D1Current=global, D1Voltage=global, Q1Current=global, Q1Voltage=global
  wires:
  Current Measurement/1 -> [CurrentSourceOutput]
  [SwitchingSignal1] -> Q1/1
  Current Measurement2/1 -> [Q1Current]
  VDiode3/1 -> [Q1Voltage]
  Current Measurement7/1 -> [D1Current]
  VDiode8/1 -> [D1Voltage]
  connections:
  VDiode3/LConn2 -- Q1/RConn1 -- Current Measurement7/LConn1 -- " RLC 5"/LConn1
  Current Measurement2/LConn1 -- In1/RConn1
  " RLC 5"/RConn1 -- " RLC 6"/LConn1
  Current Measurement/LConn1 -- " RLC 6"/RConn1
  Current Measurement2/RConn1 -- VDiode3/LConn1 -- Q1/LConn1
  Current Measurement7/RConn1 -- D1/RConn1 -- VDiode8/LConn1
  VDiode8/LConn2 -- In2/RConn1 -- Out2/RConn1 -- D1/LConn1
  Out1/RConn1 -- Current Measurement/RConn1

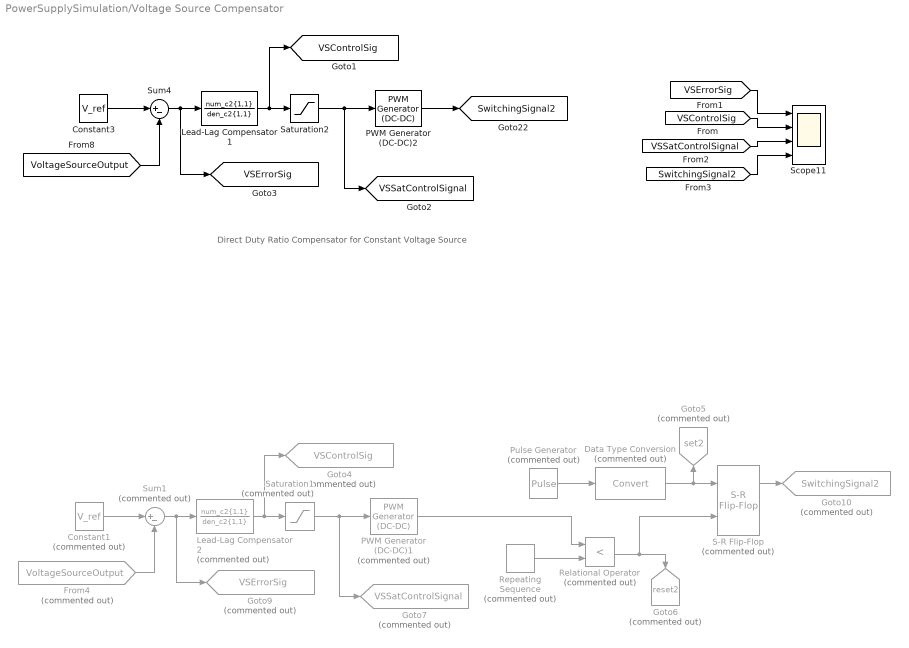
== system PowerSupplySimulation/Voltage Source Compensator ==
  note: Direct Duty Ratio Compensator for Constant Voltage Source
  Constant1 : Constant  Commented=on  Value=V_ref
  Constant3 : Constant  Value=V_ref
  Data Type Conversion : DataTypeConversion  Commented=on
  From4 : From  Commented=on  GotoTag=VoltageSourceOutput  TagVisibility=global
  Goto10 : Goto  Commented=on  GotoTag=SwitchingSignal2  TagVisibility=global
  Goto4 : Goto  Commented=on  GotoTag=VSControlSig  TagVisibility=global
  Goto5 : Goto  Commented=on  GotoTag=set2  TagVisibility=global
  Goto6 : Goto  Commented=on  GotoTag=reset2  TagVisibility=global
  Goto7 : Goto  Commented=on  GotoTag=VSSatControlSignal  TagVisibility=global
  Goto9 : Goto  Commented=on  GotoTag=VSErrorSig  TagVisibility=global
  Lead-Lag Compensator1 : TransferFcn  Numerator=num_c2{1,1}  Denominator=den_c2{1,1}
  Lead-Lag Compensator2 : TransferFcn  Commented=on  Numerator=num_c2{1,1}  Denominator=den_c2{1,1}
  PWM Generator (DC-DC)1 : powerlib_meascontrol/Pulse & Signal Generators/PWM Generator (DC-DC)  Commented=on  Fsw=f_sw  Ts=0
  PWM Generator (DC-DC)2 : powerlib_meascontrol/Pulse & Signal Generators/PWM Generator (DC-DC)  Fsw=f_sw  Ts=0
  Pulse Generator : DiscretePulseGenerator  Commented=on  PulseType=Time based  Period=1/f_sw  PulseWidth=5
  Relational Operator : RelationalOperator  Commented=on  Operator=<  OutDataTypeStr=boolean
  Repeating Sequence : simulink/Sources/Repeating Sequence  Commented=on  rep_seq_t=[0 1/f_sw]  rep_seq_y=[0 1]
  S-R Flip-Flop : simulink_extras/Flip Flops/S-R Flip-Flop  Commented=on  initial_condition=0
  Saturation1 : Saturate  Commented=on  UpperLimit=0.99  LowerLimit=0
  Saturation2 : Saturate  UpperLimit=0.99  LowerLimit=0
  Scope11 : Scope  NumInputPorts=4
  Sum1 : Sum  Commented=on  Inputs=|+-
  Sum4 : Sum  Inputs=|+-
  tag scope: SwitchingSignal2=global, VSControlSig=global, VSErrorSig=global, VSSatControlSignal=global
  wires:
  Sum4/1 -> Lead-Lag Compensator1/1, [VSErrorSig]
  Constant3/1 -> Sum4/1
  [VoltageSourceOutput] -> Sum4/2
  Lead-Lag Compensator1/1 -> [VSControlSig], Saturation2/1
  Saturation2/1 -> [VSSatControlSignal], PWM Generator (DC-DC)2/1
  PWM Generator (DC-DC)2/1 -> [SwitchingSignal2]
  [VSErrorSig] -> Scope11/1
  [SwitchingSignal2] -> Scope11/4
  [VSSatControlSignal] -> Scope11/3
  [VSControlSig] -> Scope11/2
  Pulse Generator/1 -> Data Type Conversion/1
  Data Type Conversion/1 -> S-R Flip-Flop/1, Goto5/1
  Relational Operator/1 -> S-R Flip-Flop/2, Goto6/1
  S-R Flip-Flop/1 -> Goto10/1
  PWM Generator (DC-DC)1/1 -> Relational Operator/1
  Repeating Sequence/1 -> Relational Operator/2
  Sum1/1 -> Lead-Lag Compensator2/1, Goto9/1
  Constant1/1 -> Sum1/1
  From4/1 -> Sum1/2
  Lead-Lag Compensator2/1 -> Goto4/1, Saturation1/1
  Saturation1/1 -> Goto7/1, PWM Generator (DC-DC)1/1

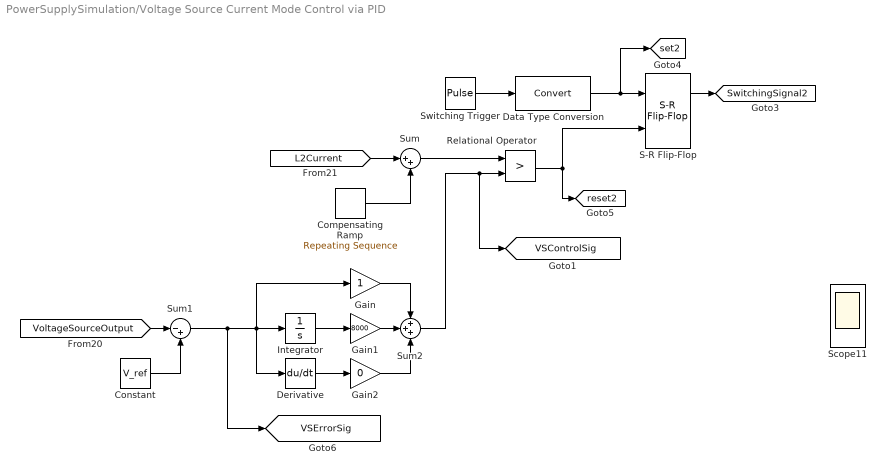
== system PowerSupplySimulation/Voltage Source Current Mode Control via PID ==
  Compensating Ramp : simulink/Sources/Repeating Sequence  rep_seq_t=[0 1/f_sw]  rep_seq_y=[0 80]
  Constant : Constant  Value=V_ref
  Data Type Conversion : DataTypeConversion
  Derivative : Derivative
  Gain : Gain
  Gain1 : Gain  Gain=8000
  Gain2 : Gain  Gain=0
  Integrator : Integrator
  Relational Operator : RelationalOperator  Operator=>  OutDataTypeStr=boolean
  S-R Flip-Flop : simulink_extras/Flip Flops/S-R Flip-Flop  initial_condition=0
  Scope11 : Scope  NumInputPorts=4
  Sum : Sum  Inputs=|++
  Sum1 : Sum  Inputs=|-+
  Sum2 : Sum  Inputs=+++
  Switching Trigger : DiscretePulseGenerator  PulseType=Time based  Period=1/f_sw  PulseWidth=5
  tag scope: SwitchingSignal2=global, VSControlSig=global, VSErrorSig=global, reset2=global, set2=global
  wires:
  Switching Trigger/1 -> Data Type Conversion/1
  Data Type Conversion/1 -> S-R Flip-Flop/1, [set2]
  Relational Operator/1 -> S-R Flip-Flop/2, [reset2]
  S-R Flip-Flop/1 -> [SwitchingSignal2]
  [L2Current] -> Sum/1
  Compensating Ramp/1 -> Sum/2
  Sum/1 -> Relational Operator/1
  [VoltageSourceOutput] -> Sum1/1
  Constant/1 -> Sum1/2
  Sum1/1 -> [VSErrorSig], Derivative/1, Gain/1, Integrator/1
  Integrator/1 -> Gain1/1
  Gain1/1 -> Sum2/2
  Gain/1 -> Sum2/1
  Sum2/1 -> [VSControlSig], Relational Operator/2
  Derivative/1 -> Gain2/1
  Gain2/1 -> Sum2/3

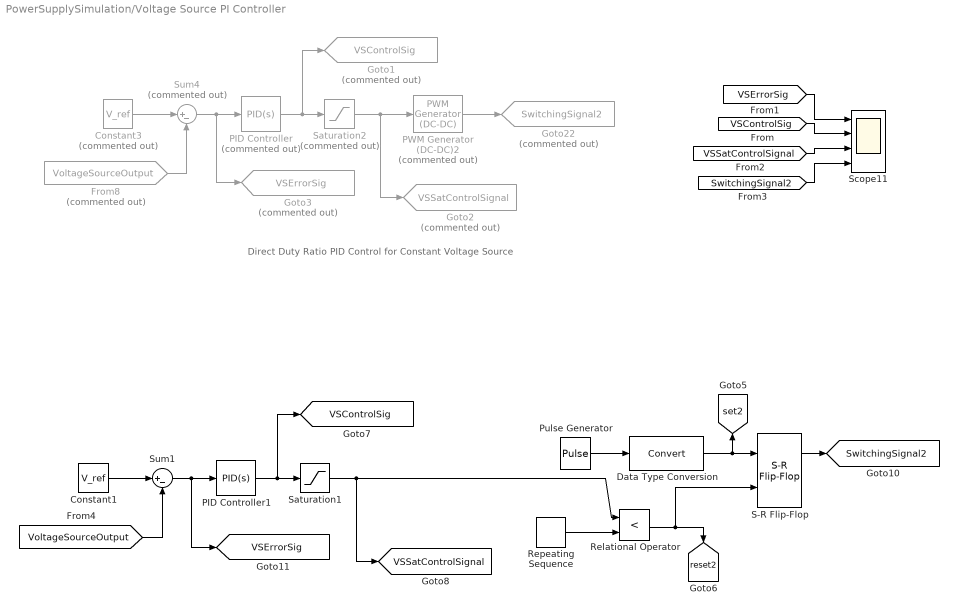
== system PowerSupplySimulation/Voltage Source PI Controller ==
  note: Direct Duty Ratio PID Control for Constant Voltage Source
  Constant1 : Constant  Value=V_ref
  Constant3 : Constant  Commented=on  Value=V_ref
  Data Type Conversion : DataTypeConversion
  From8 : From  Commented=on  GotoTag=VoltageSourceOutput  TagVisibility=global
  Goto1 : Goto  Commented=on  GotoTag=VSControlSig  TagVisibility=global
  Goto2 : Goto  Commented=on  GotoTag=VSSatControlSignal  TagVisibility=global
  Goto22 : Goto  Commented=on  GotoTag=SwitchingSignal2  TagVisibility=global
  Goto3 : Goto  Commented=on  GotoTag=VSErrorSig  TagVisibility=global
  PID Controller : simulink/Continuous/PID Controller  Commented=on  Controller=PID  TimeDomain=Continuous-time  SampleTime=-1  IntegratorMethod=Forward Euler  FilterMethod=Forward Euler  Form=Parallel  UseFilter=on  ControllerParametersSource=internal  P=2  I=0  D=0  N=0  InitialConditionSource=internal  InitialConditionForIntegrator=0  InitialConditionForFilter=0  ExternalReset=none  LimitOutput=off  UpperSaturationLimit=inf  LowerSaturationLimit=-inf  LinearizeAsGain=on  AntiWindupMode=none  Kb=1  TrackingMode=off  Kt=1  PParamMin=[]  PParamMax=[]  IParamMin=[]  IParamMax=[]  DParamMin=[]  DParamMax=[]  NParamMin=[]  NParamMax=[]  KbParamMin=[]  KbParamMax=[]  KtParamMin=[]  KtParamMax=[]  POutMin=[]  POutMax=[]  IOutMin=[]  IOutMax=[]  DOutMin=[]  DOutMax=[]  NOutMin=[]  NOutMax=[]  KbOutMin=[]  KbOutMax=[]  KtOutMin=[]  KtOutMax=[]  IntegratorOutMin=[]  IntegratorOutMax=[]  FilterOutMin=[]  FilterOutMax=[]  SumOutMin=[]  SumOutMax=[]  SumI1OutMin=[]  SumI1OutMax=[]  SumI2OutMin=[]  SumI2OutMax=[]  SumI3OutMin=[]  SumI3OutMax=[]  SumDOutMin=[]  SumDOutMax=[]  SaturationOutMin=[]  SaturationOutMax=[]  IntegratorContinuousStateAttributes=''  IntegratorStateMustResolveToSignalObject=off  IntegratorRTWStateStorageClass=Auto  FilterContinuousStateAttributes=''  FilterStateMustResolveToSignalObject=off  FilterRTWStateStorageClass=Auto  DifferentiatorICPrevScaledInput=0  DifferentiatorOutMin=[]  DifferentiatorOutMax=[]
  PID Controller1 : simulink/Continuous/PID Controller  Controller=PID  TimeDomain=Continuous-time  SampleTime=-1  IntegratorMethod=Forward Euler  FilterMethod=Forward Euler  Form=Parallel  UseFilter=on  ControllerParametersSource=internal  P=0.0189788446035745  I=203.066732311021  D=4.39436806782284e-07  N=6149446.46601847  InitialConditionSource=internal  InitialConditionForIntegrator=0  InitialConditionForFilter=0  ExternalReset=none  LimitOutput=off  UpperSaturationLimit=inf  LowerSaturationLimit=-inf  LinearizeAsGain=on  AntiWindupMode=none  Kb=1  TrackingMode=off  Kt=1  PParamMin=[]  PParamMax=[]  IParamMin=[]  IParamMax=[]  DParamMin=[]  DParamMax=[]  NParamMin=[]  NParamMax=[]  KbParamMin=[]  KbParamMax=[]  KtParamMin=[]  KtParamMax=[]  POutMin=[]  POutMax=[]  IOutMin=[]  IOutMax=[]  DOutMin=[]  DOutMax=[]  NOutMin=[]  NOutMax=[]  KbOutMin=[]  KbOutMax=[]  KtOutMin=[]  KtOutMax=[]  IntegratorOutMin=[]  IntegratorOutMax=[]  FilterOutMin=[]  FilterOutMax=[]  SumOutMin=[]  SumOutMax=[]  SumI1OutMin=[]  SumI1OutMax=[]  SumI2OutMin=[]  SumI2OutMax=[]  SumI3OutMin=[]  SumI3OutMax=[]  SumDOutMin=[]  SumDOutMax=[]  SaturationOutMin=[]  SaturationOutMax=[]  IntegratorContinuousStateAttributes=''  IntegratorStateMustResolveToSignalObject=off  IntegratorRTWStateStorageClass=Auto  FilterContinuousStateAttributes=''  FilterStateMustResolveToSignalObject=off  FilterRTWStateStorageClass=Auto  DifferentiatorICPrevScaledInput=0  DifferentiatorOutMin=[]  DifferentiatorOutMax=[]
  PWM Generator (DC-DC)2 : powerlib_meascontrol/Pulse & Signal Generators/PWM Generator (DC-DC)  Commented=on  Fsw=f_sw  Ts=0
  Pulse Generator : DiscretePulseGenerator  PulseType=Time based  Period=1/f_sw  PulseWidth=5
  Relational Operator : RelationalOperator  Operator=<  OutDataTypeStr=boolean
  Repeating Sequence : simulink/Sources/Repeating Sequence  rep_seq_t=[0 1/f_sw]  rep_seq_y=[0 1]
  S-R Flip-Flop : simulink_extras/Flip Flops/S-R Flip-Flop  initial_condition=0
  Saturation1 : Saturate  UpperLimit=0.99  LowerLimit=0
  Saturation2 : Saturate  Commented=on  UpperLimit=0.99  LowerLimit=0
  Scope11 : Scope  NumInputPorts=4
  Sum1 : Sum  Inputs=|+-
  Sum4 : Sum  Commented=on  Inputs=|+-
  tag scope: SwitchingSignal2=global, VSControlSig=global, VSErrorSig=global, VSSatControlSignal=global, reset2=global, set2=global
  wires:
  Sum4/1 -> Goto3/1, PID Controller/1
  Constant3/1 -> Sum4/1
  From8/1 -> Sum4/2
  PID Controller/1 -> Goto1/1, Saturation2/1
  Saturation2/1 -> Goto2/1, PWM Generator (DC-DC)2/1
  PWM Generator (DC-DC)2/1 -> Goto22/1
  [VSErrorSig] -> Scope11/1
  [SwitchingSignal2] -> Scope11/4
  [VSSatControlSignal] -> Scope11/3
  [VSControlSig] -> Scope11/2
  Pulse Generator/1 -> Data Type Conversion/1
  Data Type Conversion/1 -> S-R Flip-Flop/1, [set2]
  Relational Operator/1 -> S-R Flip-Flop/2, [reset2]
  S-R Flip-Flop/1 -> [SwitchingSignal2]
  Saturation1/1 -> [VSSatControlSignal], Relational Operator/1
  Sum1/1 -> [VSErrorSig], PID Controller1/1
  Constant1/1 -> Sum1/1
  [VoltageSourceOutput] -> Sum1/2
  PID Controller1/1 -> [VSControlSig], Saturation1/1
  Repeating Sequence/1 -> Relational Operator/2
